simulink model "LQT"  (R2019a)
settings: Solver=VariableStepAuto  StartTime=0.0  StopTime=100  RelTol=1e-3
values from neighbouring files (symbols this model uses):
  A1 = [X_u+X_T_u X_alpha 0 -g*cos(theta_1) ... (first row only)    [Rocket_Control_NeuroFuzzy.m]    (also in Space_Stade.m)
  B1 = [X_de ... (first row only)    [Rocket_Control_NeuroFuzzy.m]    (also in Space_Stade.m)
  C1 = [1 0 0 0 ... (first row only)    [Rocket_Control_NeuroFuzzy.m]    (also in Space_Stade.m)
  D1 = [0 ... (first row only)    [Rocket_Control_NeuroFuzzy.m]    (also in Space_Stade.m)
  Kreg = lqr(A1,B1,Q,R)    [Rocket_Control_NeuroFuzzy.m]
undefined symbols (not defined in the file or in its folder): Ke
settings Model: Creator=yuril  LastModifiedBy=yuril

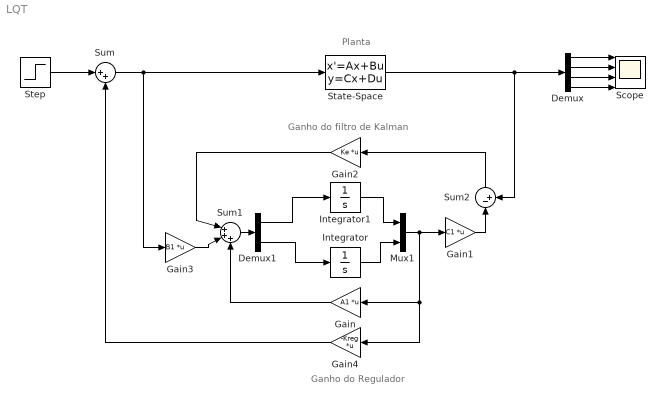
== system LQT ==
  note: Planta
  note: Ganho do filtro de Kalman
  note: Ganho do Regulador
  Demux : Demux
  Demux1 : Demux  Outputs=2
  Gain : Gain  Gain=A1  Multiplication=Matrix(K*u)
  Gain1 : Gain  Gain=C1  Multiplication=Matrix(K*u)
  Gain2 : Gain  Gain=Ke  Multiplication=Matrix(K*u)
  Gain3 : Gain  Gain=B1  Multiplication=Matrix(K*u)
  Gain4 : Gain  Gain=-Kreg  Multiplication=Matrix(K*u)
  Integrator : Integrator
  Integrator1 : Integrator
  Mux1 : Mux  Inputs=2
  Scope : Scope  NumInputPorts=4
  State-Space : StateSpace  A=A1  B=B1  C=C1  D=D1  InitialCondition=0
  Step : Step  SampleTime=0
  Sum : Sum  Inputs=|++
  Sum1 : Sum  Inputs=|+++
  Sum2 : Sum  Inputs=|-+
  wires:
  Sum/1 -> Gain3/1, State-Space/1
  State-Space/1 -> Demux/1, Sum2/2
  Sum1/1 -> Demux1/1
  Mux1/1 -> Gain4/1, Gain/1, Gain1/1
  Gain1/1 -> Sum2/1
  Demux1/1 -> Integrator1/1
  Integrator1/1 -> Mux1/1
  Demux1/2 -> Integrator/1
  Integrator/1 -> Mux1/2
  Sum2/1 -> Gain2/1
  Gain2/1 -> Sum1/1
  Gain3/1 -> Sum1/2
  Gain/1 -> Sum1/3
  Gain4/1 -> Sum/2
  Step/1 -> Sum/1
  Demux/1 -> Scope/1
  Demux/2 -> Scope/2
  Demux/3 -> Scope/3
  Demux/4 -> Scope/4
